simulink model "validation_slk_arti_d5_2015"  (Simulink 8.5)
settings: Solver=ode5  StartTime=0.0  StopTime=tf +1  FixedStep=0.005  RelTol=1e-3  AbsTol=1e-6
values from neighbouring files (symbols this model uses):
  ListePoints = [100*pi/360 100*pi/360;6*pi/360 60*pi/360]    [init_d5.m]
undefined symbols (not defined in the file or in its folder): inter_arti_d5, scarabase_ddm, scarabase_dyn
settings Model: Creator=steff  LastModifiedBy=steff  ExtModeTrigMode=oneshot  ExtModeArmWhenConnect=off
settings DataIOCC: LimitDataPoints=off  SignalLoggingName=sigsOut
settings OptimizationCC: BooleanDataType=off  ExpressionDepthLimit=128
settings DebuggingCC: SaveWithParameterizedLinksMsg=none  SignalResolutionControl=TryResolveAllWithWarning  MultiTaskDSMMsg=warning  MultiTaskCondExecSysMsg=none  FcnCallInpInsideContextMsg=EnableAllAsError  StateNameClashWarn=none  SFUnexpectedBacktrackingDiag=error  SFNoUnconditionalDefaultTransitionDiag=error
settings HardwareCC: TargetUnknown=on
settings RTWCC: TemplateMakefile=grt_vc.tmf
settings GRTTargetCC: GeneratePreprocessorConditionals=Use local settings

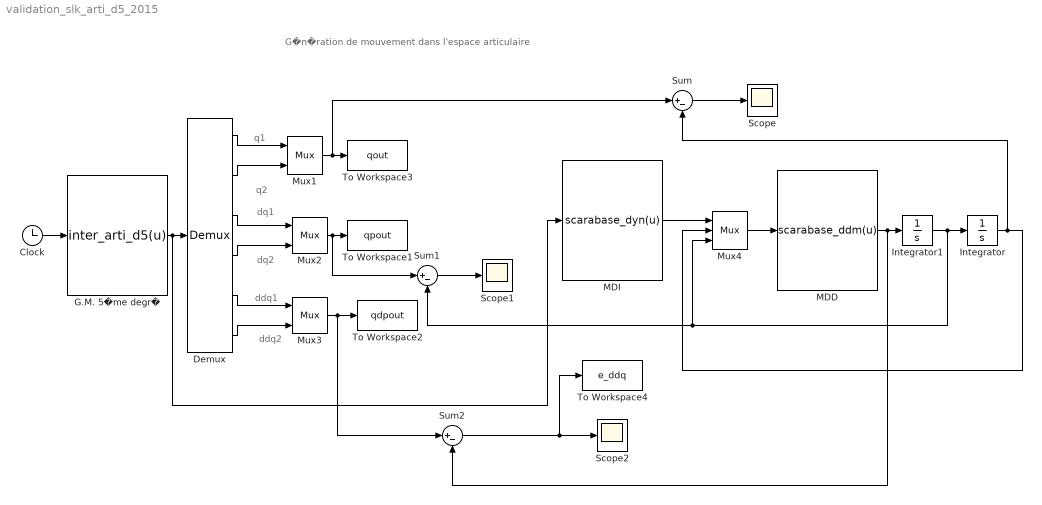
== system validation_slk_arti_d5_2015 ==
  note: G�n�ration de mouvement dans l'espace articulaire
  note: q1
  note: q2
  note: dq1
  note: dq2
  note: ddq1
  note: ddq2
  Clock : Clock
  Demux : Demux  Outputs=6
  G.M. 5�me degr� : MATLABFcn  MATLABFcn=inter_arti_d5(u)  OutputDimensions=6
  Integrator : Integrator  InitialCondition=ListePoints(1,:)
  Integrator1 : Integrator  InitialCondition=[0 0]
  MDD : MATLABFcn  MATLABFcn=scarabase_ddm(u)  OutputDimensions=2
  MDI : MATLABFcn  MATLABFcn=scarabase_dyn(u)  OutputDimensions=2  Output1D=off
  Mux1 : Mux  Inputs=2
  Mux2 : Mux  Inputs=2
  Mux3 : Mux  Inputs=2
  Mux4 : Mux  Inputs=3
  Scope : Scope
      settings: TimeRange=auto  LimitDataPoints=on  MaxDataPoints=5000  SaveToWorkspace=off  SaveName=ScopeData  YMin=-12.9945  YMax=79.21797  SampleTime=-1
  Scope1 : Scope
      settings: TimeRange=auto  LimitDataPoints=on  MaxDataPoints=5000  SaveToWorkspace=off  YMin=-0.007  YMax=0.003  SampleTime=-1
  Scope2 : Scope
      settings: TimeRange=auto  LimitDataPoints=on  MaxDataPoints=5000  SaveToWorkspace=off  SaveName=ScopeData2  YMin=-0.00001  YMax=0.00011  SampleTime=-1
  Sum : Sum  Inputs=|+-  SaturateOnIntegerOverflow=on
  Sum1 : Sum  Inputs=|+-  SaturateOnIntegerOverflow=on
  Sum2 : Sum  Inputs=|+-  SaturateOnIntegerOverflow=on
  To Workspace1 : ToWorkspace  VariableName=qpout  SampleTime=-1
  To Workspace2 : ToWorkspace  VariableName=qdpout  SampleTime=-1
  To Workspace3 : ToWorkspace  VariableName=qout  SampleTime=-1
  To Workspace4 : ToWorkspace  VariableName=e_ddq  SampleTime=-1
  wires:
  Mux2/1 -> To Workspace1/1, Sum1/1
  Clock/1 -> G.M. 5�me degr�/1
  Mux3/1 -> To Workspace2/1, Sum2/1
  G.M. 5�me degr�/1 -> Demux/1, MDI/1
  Demux/1 -> Mux1/1
  Demux/2 -> Mux1/2
  Demux/3 -> Mux2/1
  Demux/4 -> Mux2/2
  Demux/5 -> Mux3/1
  Demux/6 -> Mux3/2
  Mux1/1 -> To Workspace3/1, Sum/1
  MDD/1 -> Integrator1/1, Sum2/2
  Integrator1/1 -> Integrator/1, Mux4/3, Sum1/2
  Integrator/1 -> Mux4/2, Sum/2
  Mux4/1 -> MDD/1
  Sum/1 -> Scope/1
  MDI/1 -> Mux4/1
  Sum1/1 -> Scope1/1
  Sum2/1 -> To Workspace4/1, Scope2/1
